simulink model "sim_all"  (R2022a)
settings: Solver=FixedStepAuto  StartTime=0.0  StopTime=T  FixedStep=Ts  RelTol=1e-3
values from neighbouring files (symbols this model uses):
  A = ss_d.A    [debug_script.m]    (also in kalman_test.m; sims_all.m)
  B = ss_d.B    [debug_script.m]    (also in kalman_test.m; sims_all.m)
  C = ss_d.C    [debug_script.m]    (also in kalman_test.m; sims_all.m)
  D = ss_d.D    [debug_script.m]    (also in kalman_test.m; sims_all.m)
  freq_w = 2*pi*freq_hz    (= 1.25663706144)    [debug_script.m]    (also in sims_all.m)
  Kd = -0.5    [debug_script.m]    (also in sims_all.m)
  Ki = -0.25    [debug_script.m]    (also in sims_all.m)
  Kp = -0.3    [debug_script.m]    (also in sims_all.m)
  kx = -0.4371    [debug_script.m]    (also in sims_all.m)
  kxdot = -0.3586    [debug_script.m]    (also in sims_all.m)
  ky = -0.4371    [debug_script.m]    (also in sims_all.m)
  kydot = -0.3586    [debug_script.m]    (also in sims_all.m)
  N = 3.1722    [debug_script.m]    (also in sims_all.m)
  N_filt = 100    [sims_all.m]
  radius = 0.1    [debug_script.m]    (also in sims_all.m)
  sat_lb = -(pi/180)*5    (= -0.0872664625997)    [debug_script.m]    (also in sims_all.m)
  sat_ub = (pi/180)*5    (= 0.0872664625997)    [debug_script.m]    (also in sims_all.m)
  sys_den = sys_tf1.den{:}    [debug_script.m]    (also in sims_all.m)
  sys_num = sys_tf1.num{:}    [debug_script.m]    (also in sims_all.m)
  Ts = 0.035    [debug_script.m]    (also in kalman_test.m; sims_all.m)
  xobs0 = [0.1950;0;0.-0.1950;0]    [debug_script.m]    (also in kalman_test.m; sims_all.m)
undefined symbols (not defined in the file or in its folder): Discrete, Time
libraries: simulink_extras x4, fuzblock x3, dspfdesign x2, slpidlib x2, ctrlSharedLib x1
settings Model: Creator=michi  LastModifiedBy=michi

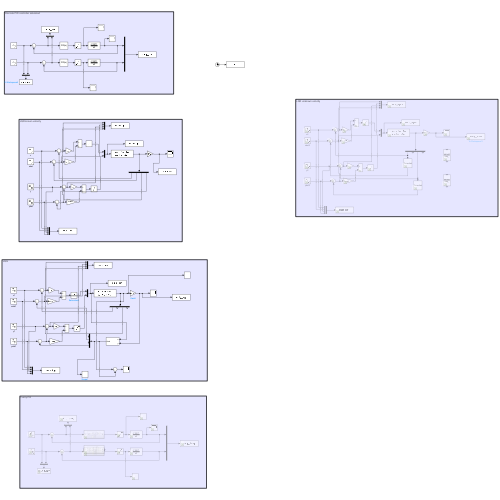
[thumbnail: Simulink's stored preview of the top-level diagram]
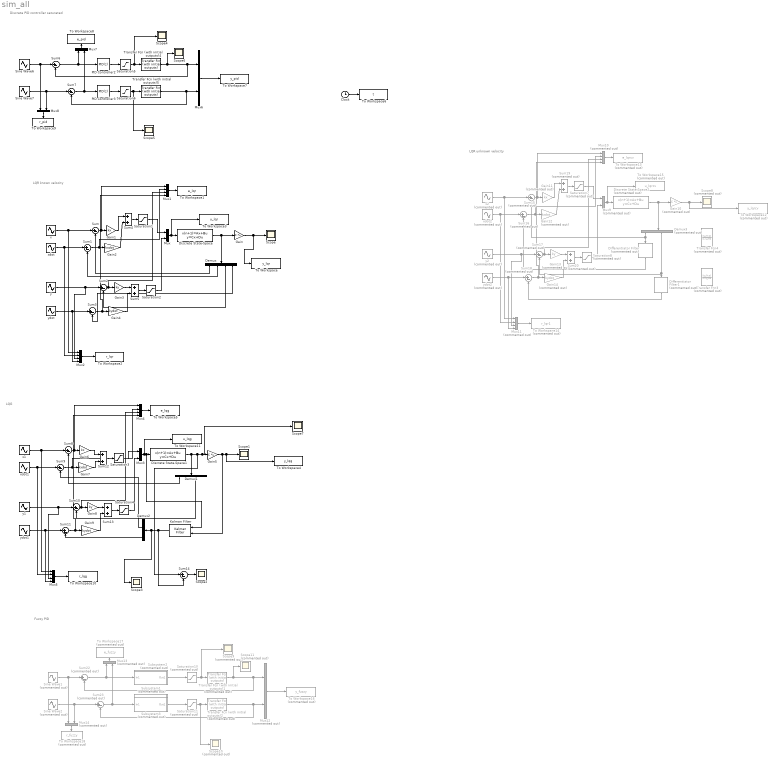
== system sim_all ==
  note: Fuzzy PID
  note: LQR known velocity
  note: Discrete PID controller saturated
  note: LQG
  note: LQR unknown velocity
  Clock : Clock
  Demux : Demux
  Demux1 : Demux
  Demux2 : Demux
  Demux3 : Demux  Commented=on
  Differentiator Filter : dspfdesign/Differentiator Filter  Commented=on  DesignForMinimumOrder=on  FilterOrder=31  PassbandRipple=0.1  ScaleCoefficients=off  SimulateUsing=Interpreted execution  roundingMode=Floor  coeffsDataTypeStr=fixdt(1,16)
      settings: SourceProductBaseCode=DS
  Differentiator Filter1 : dspfdesign/Differentiator Filter  Commented=on  DesignForMinimumOrder=on  FilterOrder=31  PassbandRipple=0.1  ScaleCoefficients=off  SimulateUsing=Interpreted execution  roundingMode=Floor  coeffsDataTypeStr=fixdt(1,16)
      settings: SourceProductBaseCode=DS
  Discrete State-Space : DiscreteStateSpace  A=A  B=B  C=eye(4)  D=zeros(4,2)  InitialCondition=[0,0,0,0]  SampleTime=-1
  Discrete State-Space1 : DiscreteStateSpace  A=A  B=B  C=eye(4)  D=zeros(4,2)  InitialCondition=[0,0,0,0]  SampleTime=-1
  Discrete State-Space2 : DiscreteStateSpace  Commented=on  A=A  B=B  C=eye(4)  D=zeros(4,2)  InitialCondition=[0,0,0,0]  SampleTime=-1
  Gain : Gain  Gain=C  Multiplication=Matrix(K*u)
  Gain1 : Gain  Gain=kx
  Gain10 : Gain  Commented=on  Gain=C  Multiplication=Matrix(K*u)
  Gain11 : Gain  Commented=on  Gain=kx
  Gain12 : Gain  Commented=on  Gain=kxdot
  Gain13 : Gain  Commented=on  Gain=ky
  Gain14 : Gain  Commented=on  Gain=kydot
  Gain2 : Gain  Gain=kxdot
  Gain3 : Gain  Gain=ky
  Gain4 : Gain  Gain=kydot
  Gain5 : Gain  Gain=C  Multiplication=Matrix(K*u)
  Gain6 : Gain  Gain=kx
  Gain7 : Gain  Gain=kxdot
  Gain8 : Gain  Gain=ky
  Gain9 : Gain  Gain=kydot
  Kalman Filter : ctrlSharedLib/Kalman Filter  TimeDomain=Discrete-Time  UseCurrentEstimator=on  ModelSource=Individual A, B, C, D matrices  ModelSourceVariable=ss(0.95,1,1,0,1)  A=A  B=B  C=C  D=D  NumberOfStates=1  NumberOfInputs=1  NumberOfOutputs=1  InitialEstimateSource=Dialog  X0=xobs0  P0=10  UseK=off  UseGH=off  NumberOfProcessNoiseInputs=1  G=1  TimeInvariantG=on  H=0  TimeInvariantH=on  Q=[1,0,0,0;0,2,0,0;0,0,1,0;0,0,0,2]  TimeInvariantQ=on  R=[1,0;0,1]  TimeInvariantR=on  N=0  TimeInvariantN=on  AddInputPort=on  AddEnablePort=off  OutputEstimatedY=off  OutputP=off  Ts=-1
  Mux{,3,6..8} (5 alike) : Mux  Inputs=2
  Mux{1..2,4..5} (4 alike) : Mux
  Mux10 : Mux  Commented=on
  Mux11 : Mux  Commented=on
  Mux{9,12..14} (4 alike) : Mux  Commented=on  Inputs=2
  PID Controller2 : slpidlib/PID Controller  Controller=PID  Form=Parallel  TimeDomain=Discrete-time  UseExternalTs=off  SampleTime=Ts  IntegratorMethod=Forward Euler  FilterMethod=Forward Euler  ControllerParametersSource=internal  P=Kp  I=Ki  UseKiTs=off  D=Kd  N=N  UseFilter=on  TunerSelectOption=Transfer Function Based (PID Tuner App)  InitialConditionSource=internal  InitialConditionForIntegrator=0  InitialConditionForFilter=0  DifferentiatorICPrevScaledInput=0  ExternalReset=none  TrackingMode=off  Kt=1  LimitOutput=off  SatLimitsSource=internal  UpperSaturationLimit=inf  LowerSaturationLimit=-inf  LinearizeAsGain=on  AntiWindupMode=none  Kb=1  POutMin=[]  POutMax=[]  IOutMin=[]  IOutMax=[]  DOutMin=[]  DOutMax=[]  NOutMin=[]  NOutMax=[]  SumOutMin=[]  SumOutMax=[]  SaturationOutMin=[]  SaturationOutMax=[]  PParamMin=[]  PParamMax=[]  IParamMin=[]  IParamMax=[]  DParamMin=[]  DParamMax=[]  NParamMin=[]  NParamMax=[]  KbParamMin=[]  KbParamMax=[]  KtParamMin=[]  KtParamMax=[]  KbOutMin=[]  KbOutMax=[]  KtOutMin=[]  KtOutMax=[]  IntegratorOutMin=[]  IntegratorOutMax=[]  FilterOutMin=[]  FilterOutMax=[]  SumI1OutMin=[]  SumI1OutMax=[]  SumI2OutMin=[]  SumI2OutMax=[]  SumI3OutMin=[]  SumI3OutMax=[]  SumI4OutMin=[]  SumI4OutMax=[]  SumDOutMin=[]  SumDOutMax=[]  DifferentiatorOutMin=[]  DifferentiatorOutMax=[]  FilterDiffOutCoefMin=[]  FilterDiffOutCoefMax=[]  ReciprocalOutMin=[]  ReciprocalOutMax=[]  SumDenOutMin=[]  SumDenOutMax=[]  SumNumOutMin=[]  SumNumOutMax=[]  DivideOutMin=[]  DivideOutMax=[]  UdiffTsProdOutMin=[]  UdiffTsProdOutMax=[]  NTsProdOutMin=[]  NTsProdOutMax=[]  UintegralTsProdOutMin=[]  UintegralTsProdOutMax=[]  UngainTsProdOutMin=[]  UngainTsProdOutMax=[]  IntegratorContinuousStateAttributes=''  IntegratorStateMustResolveToSignalObject=off  IntegratorRTWStateStorageClass=Auto  FilterContinuousStateAttributes=''  FilterStateMustResolveToSignalObject=off  FilterRTWStateStorageClass=Auto  ParallelPVariant=InternalParameters  IdealPVariant=Disabled  IVariant=InternalParameters  DVariant=InternalParameters  IntegratorVariant=Discrete  SatVariant=Disabled  AWVariant=Passthrough  PCopyVariant=Disabled  TRVariant=Disabled  FdbkBlocksVariant=Forward  IdealPFdbkVariant=Disabled  SatFdbkVariant=Disabled  DerivativeFilterVariant=ForwardEulerFilter  NVariant=InternalParameters  NCopyVariant=Disabled  FilterICVariant=InternalICsFilter  IntegratorICVariant=InternalICs  ExternalResetVariant=Disabled  TRSumVariant=Passthrough  SumFdbkVariant=Disabled  SumVariant=Sum_PID  TsampFilterVariant=InternalTs  TsampNgainVariant=Passthrough  TsampIntegralVariant=Passthrough  ExternalSaturationOutDataTypeStr=Inherit: Same as second input  aMode=0
  PID Controller3 : slpidlib/PID Controller  Controller=PID  Form=Parallel  TimeDomain=Discrete-time  UseExternalTs=off  SampleTime=Ts  IntegratorMethod=Forward Euler  FilterMethod=Forward Euler  ControllerParametersSource=internal  P=Kp  I=Ki  UseKiTs=off  D=Kd  N=N  UseFilter=on  TunerSelectOption=Transfer Function Based (PID Tuner App)  InitialConditionSource=internal  InitialConditionForIntegrator=0  InitialConditionForFilter=0  DifferentiatorICPrevScaledInput=0  ExternalReset=none  TrackingMode=off  Kt=1  LimitOutput=off  SatLimitsSource=internal  UpperSaturationLimit=inf  LowerSaturationLimit=-inf  LinearizeAsGain=on  AntiWindupMode=none  Kb=1  POutMin=[]  POutMax=[]  IOutMin=[]  IOutMax=[]  DOutMin=[]  DOutMax=[]  NOutMin=[]  NOutMax=[]  SumOutMin=[]  SumOutMax=[]  SaturationOutMin=[]  SaturationOutMax=[]  PParamMin=[]  PParamMax=[]  IParamMin=[]  IParamMax=[]  DParamMin=[]  DParamMax=[]  NParamMin=[]  NParamMax=[]  KbParamMin=[]  KbParamMax=[]  KtParamMin=[]  KtParamMax=[]  KbOutMin=[]  KbOutMax=[]  KtOutMin=[]  KtOutMax=[]  IntegratorOutMin=[]  IntegratorOutMax=[]  FilterOutMin=[]  FilterOutMax=[]  SumI1OutMin=[]  SumI1OutMax=[]  SumI2OutMin=[]  SumI2OutMax=[]  SumI3OutMin=[]  SumI3OutMax=[]  SumI4OutMin=[]  SumI4OutMax=[]  SumDOutMin=[]  SumDOutMax=[]  DifferentiatorOutMin=[]  DifferentiatorOutMax=[]  FilterDiffOutCoefMin=[]  FilterDiffOutCoefMax=[]  ReciprocalOutMin=[]  ReciprocalOutMax=[]  SumDenOutMin=[]  SumDenOutMax=[]  SumNumOutMin=[]  SumNumOutMax=[]  DivideOutMin=[]  DivideOutMax=[]  UdiffTsProdOutMin=[]  UdiffTsProdOutMax=[]  NTsProdOutMin=[]  NTsProdOutMax=[]  UintegralTsProdOutMin=[]  UintegralTsProdOutMax=[]  UngainTsProdOutMin=[]  UngainTsProdOutMax=[]  IntegratorContinuousStateAttributes=''  IntegratorStateMustResolveToSignalObject=off  IntegratorRTWStateStorageClass=Auto  FilterContinuousStateAttributes=''  FilterStateMustResolveToSignalObject=off  FilterRTWStateStorageClass=Auto  ParallelPVariant=InternalParameters  IdealPVariant=Disabled  IVariant=InternalParameters  DVariant=InternalParameters  IntegratorVariant=Discrete  SatVariant=Disabled  AWVariant=Passthrough  PCopyVariant=Disabled  TRVariant=Disabled  FdbkBlocksVariant=Forward  IdealPFdbkVariant=Disabled  SatFdbkVariant=Disabled  DerivativeFilterVariant=ForwardEulerFilter  NVariant=InternalParameters  NCopyVariant=Disabled  FilterICVariant=InternalICsFilter  IntegratorICVariant=InternalICs  ExternalResetVariant=Disabled  TRSumVariant=Passthrough  SumFdbkVariant=Disabled  SumVariant=Sum_PID  TsampFilterVariant=InternalTs  TsampNgainVariant=Passthrough  TsampIntegralVariant=Passthrough  ExternalSaturationOutDataTypeStr=Inherit: Same as second input  aMode=0
  Saturation{1..6} (6 alike) : Saturate  UpperLimit=sat_ub  LowerLimit=sat_lb
  Saturation{7..8,10..11} (4 alike) : Saturate  Commented=on  UpperLimit=sat_ub  LowerLimit=sat_lb
  Scope{,1..7} (8 alike) : Scope
  Scope{8..11} (4 alike) : Scope  Commented=on
  Sine Wave1 : Sin  Commented=on  Amplitude=radius  Frequency=freq_w  Phase=pi/2  SampleTime=Ts
  Sine Wave2 : Sin  Commented=on  Amplitude=radius  Frequency=freq_w  SampleTime=Ts
  Sine Wave6 : Sin  Amplitude=radius  Frequency=freq_w  Phase=pi/2  SampleTime=Ts
  Sine Wave7 : Sin  Amplitude=radius  Frequency=freq_w  SampleTime=Ts
  Subsystem1 : Subsystem  Commented=on
  Subsystem2 : Subsystem  Commented=on
  Subsystem3 : Subsystem  Commented=on
  Sum{,1..3,6..11,14} (11 alike) : Sum  Inputs=|+-
  Sum{4..5,12..13} (4 alike) : Sum
  Sum{15..18,22..23} (6 alike) : Sum  Commented=on  Inputs=|+-
  Sum19 : Sum  Commented=on
  Sum20 : Sum  Commented=on
  To Workspace : ToWorkspace  VariableName=y_lqr  SampleTime=-1
  To Workspace1 : ToWorkspace  VariableName=e_lqr  SampleTime=-1
  To Workspace10 : ToWorkspace  VariableName=r_lqg  SampleTime=-1
  To Workspace11 : ToWorkspace  VariableName=u_lqg  SampleTime=-1
  To Workspace12 : ToWorkspace  Commented=on  VariableName=y_lqrcv  SampleTime=-1
  To Workspace13 : ToWorkspace  Commented=on  VariableName=e_lqrcv  SampleTime=-1
  To Workspace14 : ToWorkspace  Commented=on  VariableName=r_lqr1  SampleTime=-1
  To Workspace15 : ToWorkspace  Commented=on  VariableName=u_lqrcv  SampleTime=-1
  To Workspace16 : ToWorkspace  Commented=on  VariableName=y_fuzzy  SampleTime=-1
  To Workspace17 : ToWorkspace  Commented=on  VariableName=e_fuzzy  SampleTime=-1
  To Workspace18 : ToWorkspace  Commented=on  VariableName=r_fuzzy  SampleTime=-1
  To Workspace2 : ToWorkspace  VariableName=r_lqr  SampleTime=-1
  To Workspace3 : ToWorkspace  VariableName=u_lqr  SampleTime=-1
  To Workspace4 : ToWorkspace  VariableName=y_lqg  SampleTime=-1
  To Workspace5 : ToWorkspace  VariableName=e_lqg  SampleTime=-1
  To Workspace6 : ToWorkspace  VariableName=t  SampleTime=-1
  To Workspace7 : ToWorkspace  VariableName=y_pid  SampleTime=-1
  To Workspace8 : ToWorkspace  VariableName=e_pid  SampleTime=-1
  To Workspace9 : ToWorkspace  VariableName=r_pid  SampleTime=-1
  Transfer Fcn (with initial outputs)1 : simulink_extras/Additional Linear/Transfer Fcn (with initial outputs)  Commented=on  N=sys_num  D=sys_den  Y0=init_x  U0=0
  Transfer Fcn (with initial outputs)2 : simulink_extras/Additional Linear/Transfer Fcn (with initial outputs)  Commented=on  N=sys_num  D=sys_den  Y0=init_y  U0=0
  Transfer Fcn (with initial outputs)4 : simulink_extras/Additional Linear/Transfer Fcn (with initial outputs)  N=sys_num  D=sys_den  Y0=init_x  U0=0
  Transfer Fcn (with initial outputs)5 : simulink_extras/Additional Linear/Transfer Fcn (with initial outputs)  N=sys_num  D=sys_den  Y0=init_y  U0=0
  Transfer Fcn3 : TransferFcn  Commented=on  Numerator=[N_filt 0]  Denominator=[1 N_filt]
  Transfer Fcn4 : TransferFcn  Commented=on  Numerator=[N_filt 0]  Denominator=[1 N_filt]
  x : Sin  Amplitude=radius  Frequency=freq_w  Phase=pi/2  SampleTime=Ts
  x1 : Sin  Amplitude=radius  Frequency=freq_w  Phase=pi/2  SampleTime=Ts
  x2 : Sin  Commented=on  Amplitude=radius  Frequency=freq_w  Phase=pi/2  SampleTime=Ts
  xdot : Sin  Amplitude=radius  Frequency=freq_w  SampleTime=Ts
  xdot1 : Sin  Amplitude=radius  Frequency=freq_w  SampleTime=Ts
  xdot2 : Sin  Commented=on  Amplitude=radius  Frequency=freq_w  SampleTime=Ts
  y : Sin  Amplitude=radius  Frequency=freq_w  SampleTime=Ts
  y1 : Sin  Amplitude=radius  Frequency=freq_w  SampleTime=Ts
  y2 : Sin  Commented=on  Amplitude=radius  Frequency=freq_w  SampleTime=Ts
  ydot : Sin  Amplitude=radius  Frequency=freq_w  Phase=-pi/2  SampleTime=Ts
  ydot1 : Sin  Amplitude=radius  Frequency=freq_w  Phase=-pi/2  SampleTime=Ts
  ydot2 : Sin  Commented=on  Amplitude=radius  Frequency=freq_w  Phase=-pi/2  SampleTime=Ts
  wires:
  Sine Wave7/1 -> Sum7/1, Mux8/2
  PID Controller3/1 -> Saturation6/1
  Transfer Fcn (with initial outputs)5/1 -> Sum7/2, Mux6/2
  Sum6/1 -> PID Controller2/1, Mux7/1
  Transfer Fcn (with initial outputs)4/1 -> Sum6/2, Mux6/1, Scope6/1
  Sum7/1 -> PID Controller3/1, Mux7/2
  Saturation5/1 -> Scope4/1, Transfer Fcn (with initial outputs)4/1
  Mux6/1 -> To Workspace7/1
  Saturation6/1 -> Scope5/1, Transfer Fcn (with initial outputs)5/1
  Mux8/1 -> To Workspace9/1
  PID Controller2/1 -> Saturation5/1
  Clock/1 -> To Workspace6/1
  Mux7/1 -> To Workspace8/1
  Sine Wave6/1 -> Sum6/1, Mux8/1
  Discrete State-Space/1 -> Demux/1, Gain/1
  x/1 -> Sum/1, Mux2/1
  xdot/1 -> Sum1/1, Mux2/2
  y/1 -> Mux2/3, Sum2/1
  ydot/1 -> Sum3/1, Mux2/4
  Sum2/1 -> Gain3/1, Mux1/3
  Sum3/1 -> Mux1/4, Gain4/1
  Sum4/1 -> Saturation1/1
  Gain/1 -> To Workspace/1, Scope/1
  Mux/1 -> To Workspace3/1, Discrete State-Space/1
  Demux/1 -> Sum/2
  Demux/3 -> Sum2/2
  Sum/1 -> Mux1/1, Gain1/1
  Sum1/1 -> Mux1/2, Gain2/1
  Gain1/1 -> Sum4/1
  Gain2/1 -> Sum4/2
  Saturation1/1 -> Mux/1
  Gain3/1 -> Sum5/1
  Gain4/1 -> Sum5/2
  Sum5/1 -> Saturation2/1
  Saturation2/1 -> Mux/2
  Mux1/1 -> To Workspace1/1
  Mux2/1 -> To Workspace2/1
  Sum13/1 -> Saturation4/1
  Gain9/1 -> Sum13/2
  Gain8/1 -> Sum13/1
  Sum11/1 -> Mux4/4, Gain9/1
  Gain6/1 -> Sum12/1
  Sum10/1 -> Gain8/1, Mux4/3
  y1/1 -> Mux5/3, Sum10/1
  x1/1 -> Sum8/1, Mux5/1
  Sum12/1 -> Saturation3/1
  ydot1/1 -> Sum11/1, Mux5/4
  xdot1/1 -> Sum9/1, Mux5/2
  Mux4/1 -> To Workspace5/1
  Mux3/1 -> To Workspace11/1, Kalman Filter/1, Discrete State-Space1/1
  Sum9/1 -> Mux4/2, Gain7/1
  Mux5/1 -> To Workspace10/1
  Sum8/1 -> Mux4/1, Gain6/1
  Gain7/1 -> Sum12/2
  Demux1/3 -> Sum10/2
  Discrete State-Space1/1 -> Sum14/1, Scope7/1, Gain5/1, Demux1/1
  Gain5/1 -> Kalman Filter/2, To Workspace4/1, Scope1/1
  Demux1/1 -> Sum8/2
  Demux/2 -> Sum1/2
  Demux/4 -> Sum3/2
  Kalman Filter/1 -> Scope3/1, Demux2/1, Sum14/2
  Demux2/2 -> Sum9/2
  Demux2/4 -> Sum11/2
  Sum14/1 -> Scope2/1
  Saturation8/1 -> Mux9/2
  Gain14/1 -> Sum20/2
  Gain13/1 -> Sum20/1
  Sum18/1 -> Mux10/4, Gain14/1
  Gain11/1 -> Sum19/1
  Sum20/1 -> Saturation8/1
  Sum17/1 -> Gain13/1, Mux10/3
  y2/1 -> Mux11/3, Sum17/1
  x2/1 -> Sum15/1, Mux11/1
  Saturation7/1 -> Mux9/1
  Sum19/1 -> Saturation7/1
  ydot2/1 -> Sum18/1, Mux11/4
  Gain12/1 -> Sum19/2
  xdot2/1 -> Sum16/1, Mux11/2
  Mux10/1 -> To Workspace13/1
  Mux9/1 -> To Workspace15/1, Discrete State-Space2/1
  Sum16/1 -> Mux10/2, Gain12/1
  Mux11/1 -> To Workspace14/1
  Sum15/1 -> Mux10/1, Gain11/1
  Demux3/3 -> Sum17/2, Differentiator Filter1/1
  Discrete State-Space2/1 -> Demux3/1, Gain10/1
  Gain10/1 -> To Workspace12/1, Scope8/1
  Demux3/1 -> Differentiator Filter/1, Sum15/2
  Differentiator Filter1/1 -> Sum18/2
  Differentiator Filter/1 -> Sum16/2
  Sine Wave2/1 -> Sum23/1, Mux14/2
  Subsystem3/1(Out1) -> Saturation11/1
  Mux12/1 -> To Workspace16/1
  Saturation10/1 -> Scope9/1, Transfer Fcn (with initial outputs)1/1
  Sum23/1 -> Subsystem3/1(In1), Mux13/2
  Saturation11/1 -> Scope10/1, Transfer Fcn (with initial outputs)2/1
  Mux14/1 -> To Workspace18/1
  Transfer Fcn (with initial outputs)1/1 -> Sum22/2, Mux12/1, Scope11/1
  Sum22/1 -> Subsystem2/1(In1), Mux13/1
  Transfer Fcn (with initial outputs)2/1 -> Sum23/2, Mux12/2
  Subsystem2/1(Out1) -> Saturation10/1
  Sine Wave1/1 -> Sum22/1, Mux14/1
  Mux13/1 -> To Workspace17/1
  Saturation3/1 -> Mux3/1
  Saturation4/1 -> Mux3/2

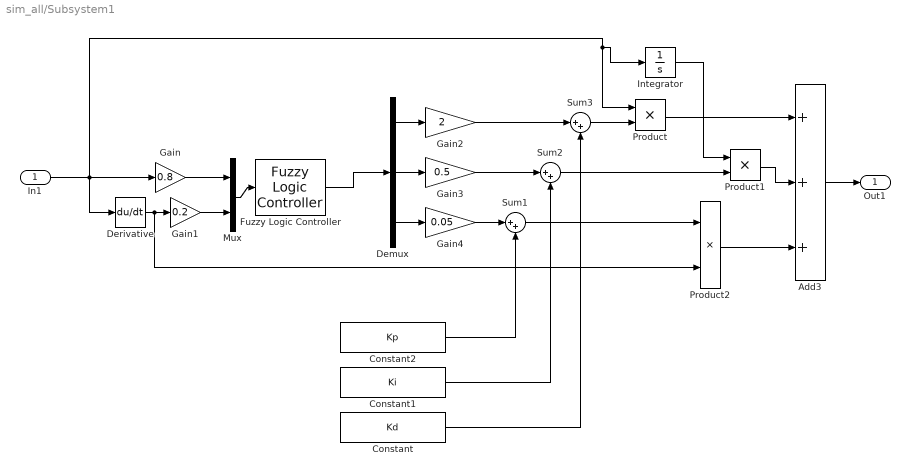
== system sim_all/Subsystem1 ==
  In1 : Inport
  Add3 : Sum  Inputs=+++
  Constant : Constant  Value=Kd
  Constant1 : Constant  Value=Ki
  Constant2 : Constant  Value=Kp
  Demux : Demux  Outputs=3
  Derivative : Derivative
  Fuzzy Logic Controller : fuzblock/Fuzzy Logic  Controller  FIS='fuzzy2.fis'  OutputSampleNumber=101  DataType=double  FuzzifiedInputs=off  RuleFiringStrengths=off  RuleOutputs=off  AggregatedOutputs=off  SimulateUsing=Interpreted execution  OutOfRangeInputValueMessage=warning  NoRuleFiredMessage=warning  EmptyOutputFuzzySetMessage=warning
  Gain : Gain  Gain=0.8
  Gain1 : Gain  Gain=0.2
  Gain2 : Gain  Gain=2
  Gain3 : Gain  Gain=0.5
  Gain4 : Gain  Gain=0.05
  Integrator : Integrator
  Mux : Mux  Inputs=2
  Product : Product
  Product1 : Product
  Product2 : Product
  Sum1 : Sum  Inputs=|++  InputSameDT=on  SaturateOnIntegerOverflow=on  OutDataTypeStr=Inherit: Same as first input
  Sum2 : Sum  Inputs=|++  InputSameDT=on  SaturateOnIntegerOverflow=on  OutDataTypeStr=Inherit: Same as first input
  Sum3 : Sum  Inputs=|++  InputSameDT=on  SaturateOnIntegerOverflow=on  OutDataTypeStr=Inherit: Same as first input
  Out1 : Outport
  wires:
  Derivative/1 -> Gain1/1, Product2/2
  Product1/1 -> Add3/2
  Constant/1 -> Sum3/2
  Demux/3 -> Gain4/1
  In1/1 -> Gain/1, Derivative/1, Integrator/1, Product/1
  Mux/1 -> Fuzzy Logic Controller/1
  Gain/1 -> Mux/1
  Integrator/1 -> Product1/1
  Add3/1 -> Out1/1
  Gain1/1 -> Mux/2
  Fuzzy Logic Controller/1 -> Demux/1
  Demux/2 -> Gain3/1
  Product2/1 -> Add3/3
  Product/1 -> Add3/1
  Demux/1 -> Gain2/1
  Constant1/1 -> Sum2/2
  Gain4/1 -> Sum1/1
  Gain3/1 -> Sum2/1
  Sum1/1 -> Product2/1
  Constant2/1 -> Sum1/2
  Sum2/1 -> Product1/2
  Sum3/1 -> Product/2
  Gain2/1 -> Sum3/1

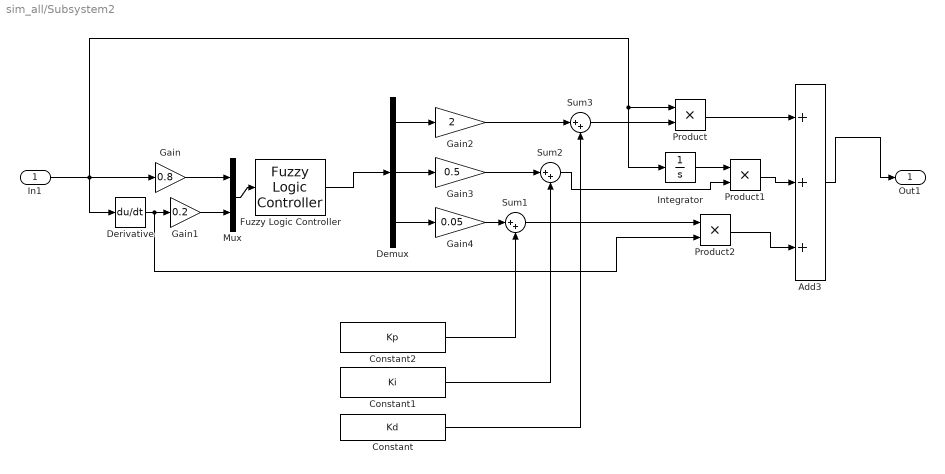
== system sim_all/Subsystem2 ==
  In1 : Inport
  Add3 : Sum  Inputs=+++
  Constant : Constant  Value=Kd
  Constant1 : Constant  Value=Ki
  Constant2 : Constant  Value=Kp
  Demux : Demux  Outputs=3
  Derivative : Derivative
  Fuzzy Logic Controller : fuzblock/Fuzzy Logic  Controller  FIS='fuzzy2.fis'  OutputSampleNumber=101  DataType=double  FuzzifiedInputs=off  RuleFiringStrengths=off  RuleOutputs=off  AggregatedOutputs=off  SimulateUsing=Interpreted execution  OutOfRangeInputValueMessage=warning  NoRuleFiredMessage=warning  EmptyOutputFuzzySetMessage=warning
  Gain : Gain  Gain=0.8
  Gain1 : Gain  Gain=0.2
  Gain2 : Gain  Gain=2
  Gain3 : Gain  Gain=0.5
  Gain4 : Gain  Gain=0.05
  Integrator : Integrator
  Mux : Mux  Inputs=2
  Product : Product
  Product1 : Product
  Product2 : Product
  Sum1 : Sum  Inputs=|++  InputSameDT=on  SaturateOnIntegerOverflow=on  OutDataTypeStr=Inherit: Same as first input
  Sum2 : Sum  Inputs=|++  InputSameDT=on  SaturateOnIntegerOverflow=on  OutDataTypeStr=Inherit: Same as first input
  Sum3 : Sum  Inputs=|++  InputSameDT=on  SaturateOnIntegerOverflow=on  OutDataTypeStr=Inherit: Same as first input
  Out1 : Outport
  wires:
  Gain2/1 -> Sum3/1
  Sum3/1 -> Product/2
  Sum2/1 -> Product1/2
  Constant2/1 -> Sum1/2
  Sum1/1 -> Product2/1
  Gain3/1 -> Sum2/1
  Gain4/1 -> Sum1/1
  Constant1/1 -> Sum2/2
  Demux/1 -> Gain2/1
  Product/1 -> Add3/1
  Product2/1 -> Add3/3
  Demux/2 -> Gain3/1
  Fuzzy Logic Controller/1 -> Demux/1
  Gain1/1 -> Mux/2
  Add3/1 -> Out1/1
  Integrator/1 -> Product1/1
  Gain/1 -> Mux/1
  Mux/1 -> Fuzzy Logic Controller/1
  In1/1 -> Integrator/1, Product/1, Derivative/1, Gain/1
  Demux/3 -> Gain4/1
  Constant/1 -> Sum3/2
  Product1/1 -> Add3/2
  Derivative/1 -> Product2/2, Gain1/1

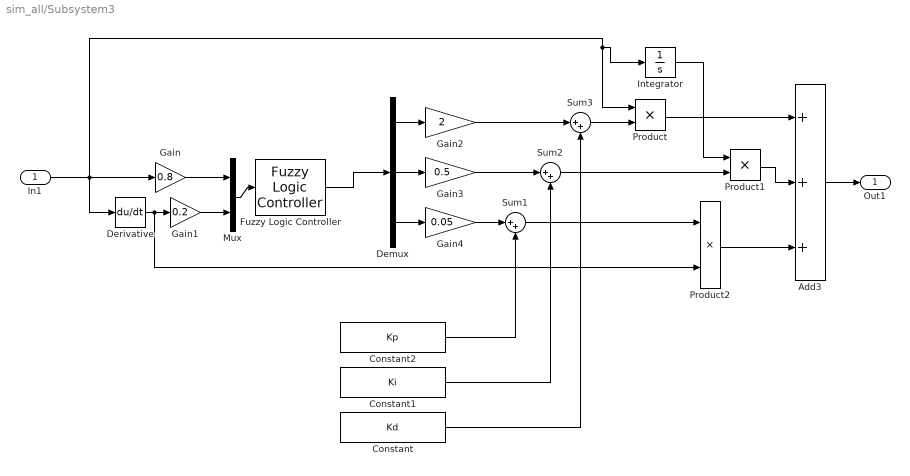
== system sim_all/Subsystem3 ==
  In1 : Inport
  Add3 : Sum  Inputs=+++
  Constant : Constant  Value=Kd
  Constant1 : Constant  Value=Ki
  Constant2 : Constant  Value=Kp
  Demux : Demux  Outputs=3
  Derivative : Derivative
  Fuzzy Logic Controller : fuzblock/Fuzzy Logic  Controller  FIS='fuzzy2.fis'  OutputSampleNumber=101  DataType=double  FuzzifiedInputs=off  RuleFiringStrengths=off  RuleOutputs=off  AggregatedOutputs=off  SimulateUsing=Interpreted execution  OutOfRangeInputValueMessage=warning  NoRuleFiredMessage=warning  EmptyOutputFuzzySetMessage=warning
  Gain : Gain  Gain=0.8
  Gain1 : Gain  Gain=0.2
  Gain2 : Gain  Gain=2
  Gain3 : Gain  Gain=0.5
  Gain4 : Gain  Gain=0.05
  Integrator : Integrator
  Mux : Mux  Inputs=2
  Product : Product
  Product1 : Product
  Product2 : Product
  Sum1 : Sum  Inputs=|++  InputSameDT=on  SaturateOnIntegerOverflow=on  OutDataTypeStr=Inherit: Same as first input
  Sum2 : Sum  Inputs=|++  InputSameDT=on  SaturateOnIntegerOverflow=on  OutDataTypeStr=Inherit: Same as first input
  Sum3 : Sum  Inputs=|++  InputSameDT=on  SaturateOnIntegerOverflow=on  OutDataTypeStr=Inherit: Same as first input
  Out1 : Outport
  wires:
  Gain2/1 -> Sum3/1
  Sum3/1 -> Product/2
  Sum2/1 -> Product1/2
  Constant2/1 -> Sum1/2
  Sum1/1 -> Product2/1
  Gain3/1 -> Sum2/1
  Gain4/1 -> Sum1/1
  Constant1/1 -> Sum2/2
  Demux/1 -> Gain2/1
  Product/1 -> Add3/1
  Product2/1 -> Add3/3
  Demux/2 -> Gain3/1
  Fuzzy Logic Controller/1 -> Demux/1
  Gain1/1 -> Mux/2
  Add3/1 -> Out1/1
  Integrator/1 -> Product1/1
  Gain/1 -> Mux/1
  Mux/1 -> Fuzzy Logic Controller/1
  In1/1 -> Product/1, Integrator/1, Derivative/1, Gain/1
  Demux/3 -> Gain4/1
  Constant/1 -> Sum3/2
  Product1/1 -> Add3/2
  Derivative/1 -> Product2/2, Gain1/1
